simulink model "Clark_Park"  (R2020b)
settings: Solver=ode45  StartTime=0.0  StopTime=0.1  RelTol=1e-3  EnableMultiTasking=on
undefined symbols (not defined in the file or in its folder): DiscIntNeverNeededParam
settings Model: Creator=Lei  LastModifiedBy=Ray
settings DataIOCC: LimitDataPoints=on  SaveFormat=Array  ReturnWorkspaceOutputs=off
settings OptimizationCC: LifeSpan=inf
settings DebuggingCC: SolverPrmCheckMsg=warning  SFUnexpectedBacktrackingDiag=warning  SFNoUnconditionalDefaultTransitionDiag=warning  SFExecutionAtInitializationDiag=none  ArithmeticOperatorsInVariantConditions=warning
settings HardwareCC: ProdBitPerPointer=32  ProdBitPerSizeT=32  ProdBitPerPtrDiffT=32  ProdLargestAtomicFloat=None  ProdIntDivRoundTo=Undefined  ProdEndianess=Unspecified  ProdWordSize=32  ProdHWDeviceType=32-bit Generic
settings ModelReferenceCC: PropagateSignalLabelsOutOfModel=off
settings SFSimCC: SimUseLocalCustomCode=off  CustomCodeUndefinedFunction=UseInterfaceOnly
settings RTWCC: RTWUseLocalCustomCode=off
settings CodeAppCC: StateflowObjectComments=on
settings GRTTargetCC: TargetLangStandard=C89/C90 (ANSI)
settings ConfigComp: CovMetricSettings=dw  CovSaveCumulativeToWorkspaceVar=on  CovSaveSingleToWorkspaceVar=on  CovExternalEMLEnable=off  CovSFcnEnable=off

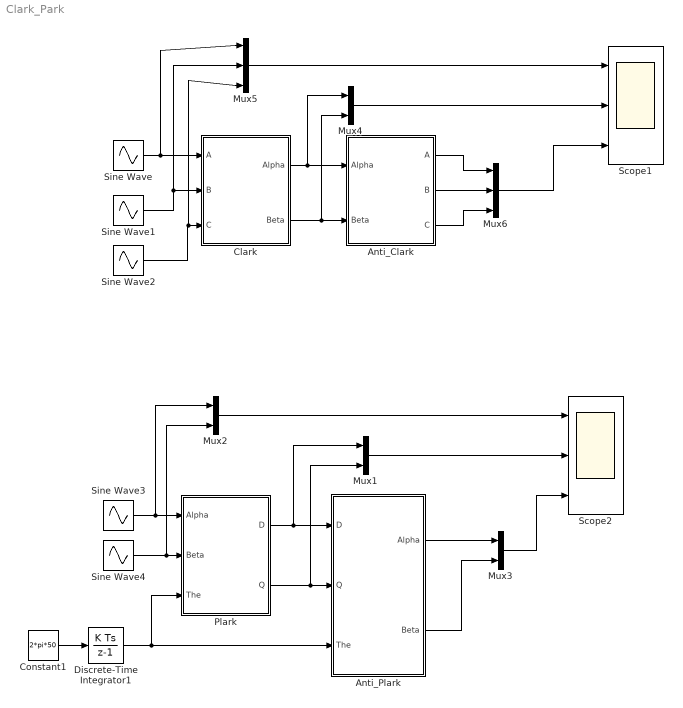
== system Clark_Park ==
  Anti_Clark : Subsystem
  Anti_Plark : Subsystem
  Clark : Subsystem
  Constant1 : Constant  Value=2*pi*50
  Discrete-Time Integrator1 : DiscreteIntegrator  SampleTime=10e-6  ICPrevOutput=DiscIntNeverNeededParam  ICPrevScaledInput=DiscIntNeverNeededParam
  Mux{1..4} (4 alike) : Mux  Inputs=2
  Mux5 : Mux  Inputs=3
  Mux6 : Mux  Inputs=3
  Plark : Subsystem
  Scope1 : Scope  NumInputPorts=3
  Scope2 : Scope  NumInputPorts=3
  Sine Wave : Sin  Amplitude=100  Frequency=2*pi*50  SampleTime=10e-6
  Sine Wave1 : Sin  Amplitude=100  Frequency=2*pi*50  Phase=-2/3*pi  SampleTime=10e-6
  Sine Wave2 : Sin  Amplitude=100  Frequency=2*pi*50  Phase=2/3*pi  SampleTime=10e-6
  Sine Wave3 : Sin  Amplitude=100  Frequency=2*pi*50  Phase=pi/2  SampleTime=10e-6
  Sine Wave4 : Sin  Amplitude=100  Frequency=2*pi*50  SampleTime=10e-6
  wires:
  Plark/2(Q) -> Mux1/2, Anti_Plark/2(Q)
  Sine Wave4/1 -> Mux2/2, Plark/2(Beta)
  Sine Wave3/1 -> Mux2/1, Plark/1(Alpha)
  Plark/1(D) -> Mux1/1, Anti_Plark/1(D)
  Constant1/1 -> Discrete-Time Integrator1/1
  Discrete-Time Integrator1/1 -> Plark/3(The), Anti_Plark/3(The)
  Anti_Plark/1(Alpha) -> Mux3/1
  Anti_Plark/2(Beta) -> Mux3/2
  Mux1/1 -> Scope2/2
  Mux2/1 -> Scope2/1
  Mux3/1 -> Scope2/3
  Clark/1(Alpha) -> Mux4/1, Anti_Clark/1(Alpha)
  Sine Wave/1 -> Mux5/1, Clark/1(A)
  Sine Wave2/1 -> Mux5/3, Clark/3(C)
  Clark/2(Beta) -> Mux4/2, Anti_Clark/2(Beta)
  Sine Wave1/1 -> Mux5/2, Clark/2(B)
  Anti_Clark/2(B) -> Mux6/2
  Anti_Clark/3(C) -> Mux6/3
  Mux4/1 -> Scope1/2
  Mux5/1 -> Scope1/1
  Anti_Clark/1(A) -> Mux6/1
  Mux6/1 -> Scope1/3

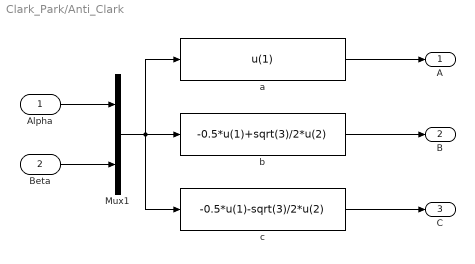
== system Clark_Park/Anti_Clark ==
  Alpha : Inport
  Beta : Inport  Port=2
  Mux1 : Mux  Inputs=2
  a : Fcn  Expr=u(1)
  b : Fcn  Expr=-0.5*u(1)+sqrt(3)/2*u(2)
  c : Fcn  Expr=-0.5*u(1)-sqrt(3)/2*u(2)
  A : Outport
  B : Outport  Port=2
  C : Outport  Port=3
  wires:
  b/1 -> B/1
  c/1 -> C/1
  Beta/1 -> Mux1/2
  Alpha/1 -> Mux1/1
  a/1 -> A/1
  Mux1/1 -> a/1, c/1, b/1

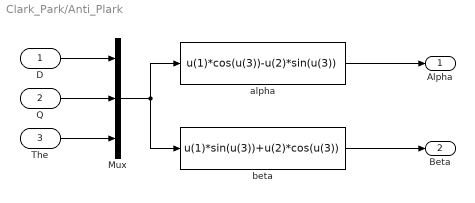
== system Clark_Park/Anti_Plark ==
  D : Inport
  Q : Inport  Port=2
  The : Inport  Port=3
  Mux : Mux  Inputs=3
  alpha : Fcn  Expr=u(1)*cos(u(3))-u(2)*sin(u(3))
  beta : Fcn  Expr=u(1)*sin(u(3))+u(2)*cos(u(3))
  Alpha : Outport
  Beta : Outport  Port=2
  wires:
  alpha/1 -> Alpha/1
  Q/1 -> Mux/2
  The/1 -> Mux/3
  D/1 -> Mux/1
  Mux/1 -> beta/1, alpha/1
  beta/1 -> Beta/1

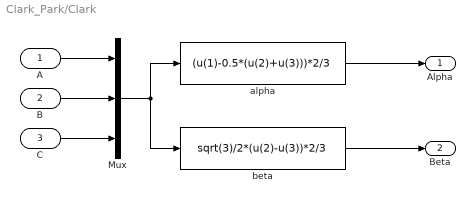
== system Clark_Park/Clark ==
  A : Inport
  B : Inport  Port=2
  C : Inport  Port=3
  Mux : Mux  Inputs=3
  alpha : Fcn  Expr=(u(1)-0.5*(u(2)+u(3)))*2/3
  beta : Fcn  Expr=sqrt(3)/2*(u(2)-u(3))*2/3
  Alpha : Outport
  Beta : Outport  Port=2
  wires:
  alpha/1 -> Alpha/1
  B/1 -> Mux/2
  C/1 -> Mux/3
  A/1 -> Mux/1
  Mux/1 -> beta/1, alpha/1
  beta/1 -> Beta/1

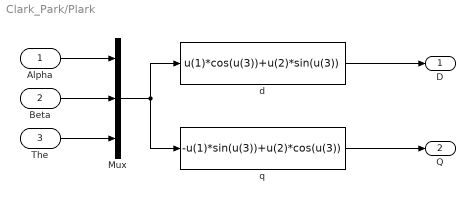
== system Clark_Park/Plark ==
  Alpha : Inport
  Beta : Inport  Port=2
  The : Inport  Port=3
  Mux : Mux  Inputs=3
  d : Fcn  Expr=u(1)*cos(u(3))+u(2)*sin(u(3))
  q : Fcn  Expr=-u(1)*sin(u(3))+u(2)*cos(u(3))
  D : Outport
  Q : Outport  Port=2
  wires:
  d/1 -> D/1
  Beta/1 -> Mux/2
  The/1 -> Mux/3
  Alpha/1 -> Mux/1
  Mux/1 -> q/1, d/1
  q/1 -> Q/1
